simulink model "PassCarModel_RL_config"  (R2024b)
settings: Solver=FixedStepAuto  StartTime=0.0  StopTime=Tf  FixedStep=.001  RelTol=1e-2
StartFcn:
  | %tic
StopFcn:
  | %toc
model workspace (MAT data in the model file):
  AverageTimeInterval = 0.5
  Downshift_Speeds = [9.5625 12.9375 16.3125 19.6875 23.0625 26.4375 29.8125 33.1875 36.5625 39.9375 43.3125 46.6875 ... (28 elements, 4x7)]
  EEC_Counter : Simulink.Parameter (value not decoded)
  EngRevLim = 7000
  FuzzOffset : Simulink.Parameter (value not decoded)
  FuzzRange : Simulink.Parameter (value not decoded)
  Fuzzing : Simulink.Parameter (value not decoded)
  Pedal_Positions = [0.1 0.4 0.5 0.9]
  TrackPoints = [0 36.336 72.672 109.008 145.344 181.68 218.016 254.352 290.688 327.024 363.36 403.196036522 ... (360 elements, 120x3)]
  Upshift_Speeds = [12.9375 16.3125 19.6875 33 26.4375 29.8125 33.1875 52.5 39.9375 43.3125 46.6875 77.25 ... (28 elements, 4x7)]
  VEH : object (value not decoded)
  gradbp : Simulink.Parameter (value not decoded)
  origin : Simulink.Parameter (value not decoded)
  rayDirections = [0 0 0 0 0 0 0 0 0 0 0 0 ... (363 elements, 121x3)]
  rayLengths = [20 20 20 20 20 20 20 20 20 20 20 20 ... (121 elements, 121x1)]
  rayOrigins = [0.5 0.4 0.3 0.2 0.1 0 -0.1 -0.2 -0.3 -0.4 -0.5 0.5 ... (363 elements, 121x3)]
  theta : Simulink.Parameter (value not decoded)
  totalDistance : Simulink.Parameter (value not decoded)
  vel_profile3 : Simulink.Parameter (value not decoded)
  xEast : Simulink.Parameter (value not decoded)
  yNorth : Simulink.Parameter (value not decoded)
symbols that are objects in the model workspace (value not decoded): gradbp, origin, theta, totalDistance, VEH, vel_profile3, xEast, yNorth
undefined symbols (not defined in the file or in its folder): DecelR, DiscIntNeverNeededParam, dspblkCoreblockFVToolHelper, FO_max, FO_min, FR_max, FR_min, gcbh, ODevR, Sim3dSensor, Ts
libraries: simulink x20, dspstat3 x8, autolibutils x6, sim3dgroundtruthsensorlib x2, rllib x1, slpidlib x1, autolibtranscontrolscommon x1, vehdynlibdriver x1, sharedtransform x1, vehdynlibviscommon x1, vehdynlibsens x1
(part 5 of 5)

== matlab function PassCarModel_RL_config/Controllers and CAN network/Controllers/Brake Pressure Control/Bang Bang ABS/Kappa/MATLAB Function ==
  data: Omega input; xdot input; KappaEst output
function KappaEst = fcn(Omega, xdot)

Re = 0.29;
KappaEst = 0;
WhlSpd = Omega * Re;

if xdot*WhlSpd ~= 0
    KappaEst = (WhlSpd - xdot)/max([abs(xdot) abs(WhlSpd)]);
end

== matlab function PassCarModel_RL_config/Controllers and CAN network/Controllers/Brake Pressure Control/Five-State ABS and TCS/Wheel Accel and Slip Estimator/Kappa/MATLAB Function ==
  data: Omega input; xdot input; KappaEst output
function KappaEst = fcn(Omega, xdot)

Re = 0.29;
KappaEst = 0;
WhlSpd = Omega * Re;

v_max = max([abs(xdot) abs(WhlSpd)]);
%if xdot*WhlSpd ~= 0
if v_max ~= 0
    KappaEst = (WhlSpd - xdot)/v_max;
end

== stateflow chart PassCarModel_RL_config/Controllers and CAN network/Controllers/Brake Pressure Control/Five-State ABS and TCS/ABSCtrlForEach/For Each Subsystem/ABSForEachWheel ==
  state ABSOff
    entry:
    PbOutput = Pref;
    Flag = 0;
    during:
    PbOutput = Pref;
  state Normal
    entry:
    PbOutput = Pref;
    Flag = 0;
    during:
    PbOutput = Pref;
  state ABSOn
    state Phase1
      entry:
      PbOutput = v1;
      Flag = 1;
    state Phase5
      entry:
      PbOutput = v5;
      Flag = 5;
    state Phase2
      entry:
      PbOutput = 0;
      Flag = 2;
    state Phase4
      entry:
      PbOutput = 0;
      Flag = 4;
    state Phase3
      entry:
      PbOutput = v4;
      Flag = 3;
    (default) -> Phase1
    Phase5 -> Phase1 : [e2 < a2]
    Phase1 -> Phase2 : [e2 >= b]
    Phase4 -> Phase5 : [e2 <= a1]
    Phase2 -> Phase3 : [e2 >= A]
    Phase3 -> Phase4 : [e2 < A]
  (default) -> ABSOff
  ABSOn -> ABSOff : [abs(VehSpd) < 0.1 || Pref <= 0]
  Normal -> ABSOff [order 2] : [Pref <= 0]
  ABSOff -> Normal : [Pref > 0 && e2 < a2]
  Normal -> ABSOn [order 1] : [e1 < 0]
  data: e1 input; e2 input; PbOutput output; Flag output; b parameter; v1 parameter; v4 parameter; v5 parameter; A parameter; a2 parameter; a1 parameter; Pref input; VehSpd input
